simulink model "uas_jury"  (R2021a)
settings: Solver=FixedStepAuto  StartTime=0.0  StopTime=Inf  FixedStep=0.04  RelTol=1e-3
model workspace: external: MAT-File (data not in the file)
libraries: robotlib x3
settings Model: EnablePacing=on  OrderedModelArguments=off  Creator=david  LastModifiedBy=david
settings SolverCC: AlgebraicLoopSolver=TrustRegion
settings DataIOCC: LimitDataPoints=on  MaxDataPoints=10000
settings OptimizationCC: EnhancedBackFolding=on  PassReuseOutputArgsThreshold=0  ZeroExternalMemoryAtStartup=off  ZeroInternalMemoryAtStartup=off  MaxStackSize=64  OptimizeBlockOrder=speed  DifferentSizesBufferReuse=on  OptimizationCustomize=off
settings DebuggingCC: ParameterTunabilityLossMsg=error  AllowSymbolicDim=off  SFUnexpectedBacktrackingDiag=warning  SFNoUnconditionalDefaultTransitionDiag=warning  SFExecutionAtInitializationDiag=none  SFMachineParentedDataDiag=warning  UnderSpecifiedDimensionMsg=warning  ArithmeticOperatorsInVariantConditions=warning
settings HardwareCC: ProdBitPerPointer=32  ProdBitPerSizeT=32  ProdBitPerPtrDiffT=32  ProdLargestAtomicFloat=None  ProdIntDivRoundTo=Undefined  ProdEndianess=Unspecified  ProdWordSize=32  ProdHWDeviceType=Generic->Unspecified (assume 32-bit Generic)  UseEmbeddedCoderFeatures=off
settings SFSimCC: SimUseLocalCustomCode=off  MATLABDynamicMemAlloc=off  CustomCodeUndefinedFunction=UseInterfaceOnly  SimTargetLang=C++
settings RTWCC: SystemTargetFile=ert.tlc  HardwareBoard=Robot Operating System (ROS)  TLCOptions="-aInlineSetEventsForThisBaseRateFcn=TLC_FALSE -aSuppressMultiTaskScheduler=TLC_FALSE  -aRateBasedStepFcn=0"  TemplateMakefile=ert_default_tmf  RTWUseLocalCustomCode=off  Toolchain=Catkin  TargetLang=C++
settings CodeAppCC: ForceParamTrailComments=on  OperatorAnnotations=on
settings ERTTargetCC: ERTCustomFileBanners=off  CodeInterfacePackaging=C++ class  SupportContinuousTime=on  SupportNonInlinedSFcns=on  RemoveResetFunc=off  ModelStepFunctionPrototypeControlCompliant=off  RootIOFormat=Structure reference
settings ConfigComp: CovMetricSettings=dw  CovSaveCumulativeToWorkspaceVar=on  CovSaveSingleToWorkspaceVar=on  CovExternalEMLEnable=off  CovSFcnEnable=off
settings SimscapeCC: SimscapeLogType=all  SimscapeLogSimulationStatistics=on  SimscapeLogDataHistory=10000

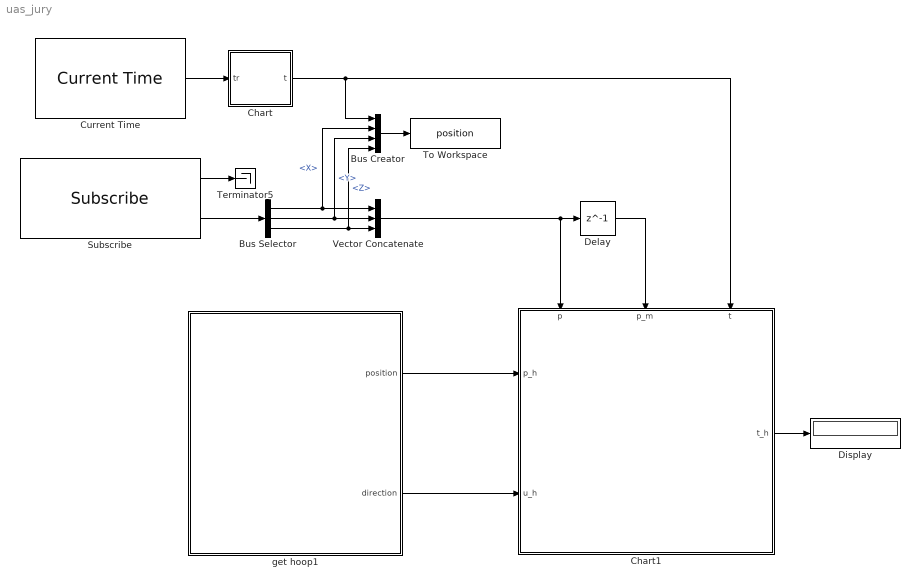
== system uas_jury ==
  Bus Creator : BusCreator  Inputs=4
  Bus Selector : BusSelector  OutputSignals=Pose.Position.X,Pose.Position.Y,Pose.Position.Z
  Chart : Stateflow chart  TreatAsAtomicUnit=on
  Chart1 : Stateflow chart  TreatAsAtomicUnit=on
      settings: PortSchema="{\"entries\":[{\"content\":{\"sides\":[{\"content\":{\"connectorIds\":[\"In1\",\"In2\"]},\"type\":\"ConnectorPlacement.EquallySpacedRectSide\",\"uuid\":\"cbe436de-a78a-4d54-ada1-ffe9c85ec4dd\"},{\"content\":{\"connectorIds\":[\"Out1\"],\"side\":\"RIGHT\"},\"type\":\"ConnectorPlacement.EquallySpacedRectSide\",\"uuid\":\"d6c18add-11e9-424c-8ba7-88879ae0fd80\"},{\"content\":{\"connectorIds\":[\"In5\",\"In4\",\"In3\"],\"side\":\"TOP\"},\"type\":\"ConnectorPlacement.EquallySpacedRectSide\",\"uuid\":\"76b9d127-0554-4e6d-8dbe-789f038cc216\"}]},\"type\":\"ConnectorPlacement.EquallySpacedConnector\",\"uuid\":\"bfa6469e-b649-49a2-8593-af73454ffe28\"}],\"packageUris\":[\"http://schema.mathworks.com/mf0/Connector/R2020b\"],\"version\":\"1.0\"}"
  Current Time : robotlib/Current Time  OutputFormat=double  SampleTime=-1  ModelName=uas_jury
      settings: SourceProductBaseCode=RR
  Delay : Delay  DelayLength=1
  Display : Display
  Subscribe : robotlib/Subscribe  topicSource=Specify your own  topic=/vrpn_client_node/cf18/pose  messageType=geometry_msgs/PoseStamped  SampleTime=-1  legacyBusStruct=off  messageQueueLength=1
  Terminator5 : Terminator
  To Workspace : ToWorkspace  VariableName=position  SaveFormat=Timeseries  SampleTime=-1
  Vector Concatenate : Concatenate  NumInputs=3  Mode=Multidimensional array
  get hoop1 : Subsystem
  wires:
  Current Time/1 -> Chart/1(tr)
  Subscribe/2 -> Bus Selector/1
  Bus Selector/2 -> Vector Concatenate/2, Bus Creator/3  "<Y>"
  Bus Selector/3 -> Vector Concatenate/3, Bus Creator/4  "<Z>"
  Bus Selector/1 -> Vector Concatenate/1, Bus Creator/2  "<X>"
  Subscribe/1 -> Terminator5/1
  Chart/1(t) -> Chart1/3(t), Bus Creator/1
  Bus Creator/1 -> To Workspace/1
  Delay/1 -> Chart1/4(p_m)
  Vector Concatenate/1 -> Chart1/5(p), Delay/1
  get hoop1/1(position) -> Chart1/1(p_h)
  get hoop1/2(direction) -> Chart1/2(u_h)
  Chart1/1(t_h) -> Display/1

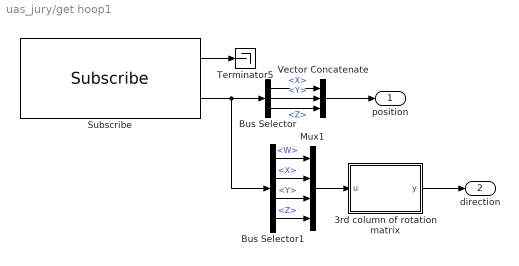
== system uas_jury/get hoop1 ==
  3rd column of rotation matrix : MATLAB Function  TreatAsAtomicUnit=on
  Bus Selector : BusSelector  OutputSignals=Pose.Position.X,Pose.Position.Y,Pose.Position.Z
  Bus Selector1 : BusSelector  OutputSignals=Pose.Orientation.W,Pose.Orientation.X,Pose.Orientation.Y,Pose.Orientation.Z
  Mux1 : Mux
  Subscribe : robotlib/Subscribe  topicSource=Specify your own  topic=/vrpn_client_node/hoop1/pose  messageType=geometry_msgs/PoseStamped  SampleTime=-1  legacyBusStruct=off  messageQueueLength=1
  Terminator5 : Terminator
  Vector Concatenate : Concatenate  NumInputs=3  Mode=Multidimensional array
  position : Outport
  direction : Outport  Port=2
  wires:
  Subscribe/2 -> Bus Selector1/1, Bus Selector/1
  Bus Selector/3 -> Vector Concatenate/3  "<Z>"
  Bus Selector/1 -> Vector Concatenate/1  "<X>"
  Bus Selector/2 -> Vector Concatenate/2  "<Y>"
  Subscribe/1 -> Terminator5/1
  Bus Selector1/1 -> Mux1/1  "<W>"
  Bus Selector1/2 -> Mux1/2  "<X>"
  Bus Selector1/3 -> Mux1/3  "<Y>"
  Bus Selector1/4 -> Mux1/4  "<Z>"
  Mux1/1 -> 3rd column of rotation matrix/1(u)
  3rd column of rotation matrix/1(y) -> direction/1
  Vector Concatenate/1 -> position/1

== stateflow chart uas_jury/Chart1 ==
  state waiting
  state done
  (default) -> waiting
  waiting -> done : [in_hoop(p_h, u_h, p, p_m)]{t_h = t}
  data: position_hoop function_input; direction_hoop function_input; position function_input; is_in_hoop function_output; previous_position function_input; p_h input; u_h input; t input; t_h output; p_m input; p input
  function is_in_hoop = in_hoop(position_hoop, direction_hoop, position, previous_position):
    | function is_in_hoop = in_hoop(position_hoop, direction_hoop, position, previous_position)
    | p_B_H = position - position_hoop;
    | p_Bm_H = previous_position - position_hoop;
    | c1 = norm(p_B_H, 2) < 0.1;
    | c2 = norm(p_Bm_H, 2) < 0.1;
    | c3 = direction_hoop.' * p_B_H > 0;
    | c4 = direction_hoop.' * p_Bm_H > 0;
    | is_in_hoop = c1 && c2 && xor(c3, c4);
    | end

== matlab function uas_jury/get hoop1/3rd column of rotation matrix ==
  data: u input size=[1 4]; y output size=[3 1]
function y = get_r3(u)

R = quat2rotm(u);

y = R(:,3);

== stateflow chart uas_jury/Chart ==
  state run
    t = tr - t0
  (default) -> run : {t0 = tr}
  data: t output; t0 local; tr input
